simulink model "schemat_8"  (R2020a)
settings: Solver=VariableStepAuto  StartTime=0.0  StopTime=10.0  RelTol=1e-3
values from neighbouring files (symbols this model uses):
  dfwe1 = 0    [gotowe2.m]    (also in lab7.m; lab8.m = 0.5)
  dfwe2 = 0.1*fwemax    (= 0.5)    [gotowe2.m]    (also in lab7.m = 0; lab8.m = 0)
  G11a = A2    (= 10)    [gotowe2.m]    (also in lab8.m)
  G11b = a1+a2    (= 15)    [gotowe2.m]    (also in lab8.m)
  G12 = a1    (= 10)    [gotowe2.m]    (also in lab8.m)
  G21 = a1    (= 10)    [gotowe2.m]    (also in lab8.m)
  G22a = A1    (= 10)    [gotowe2.m]    (also in lab8.m)
  G22b = a1    (= 10)    [gotowe2.m]    (also in lab8.m)
  h10 = (fwe1/a1)+h20    (= 0.8)    [gotowe2.m]    (also in lab7.m = 0.2; lab8.m = (fwe1/a1)+h20)
  h20 = (fwe1+fwe2)/(a2)    (= 0.7)    [gotowe2.m]    (also in lab7.m = 0.2; lab8.m = (fwe1+fwe2)/(a2))
  M1 = A1*A2    (= 100)    [gotowe2.m]    (also in lab8.m)
  M2 = A1*a1+A1*a2+a1*A2    (= 250)    [gotowe2.m]    (also in lab8.m)
  M3 = a1*a2    (= 50)    [gotowe2.m]    (also in lab8.m)
settings Model: Creator=pc  LastModifiedBy=pc

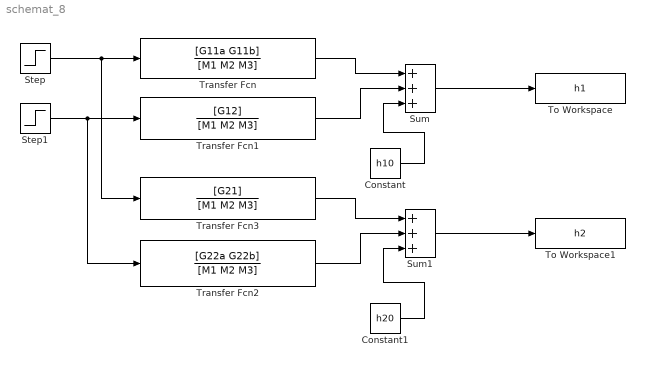
== system schemat_8 ==
  Constant : Constant  Value=h10
  Constant1 : Constant  Value=h20
  Step : Step  Time=5  After=0+dfwe1  SampleTime=0
  Step1 : Step  Time=5  After=0+dfwe2  SampleTime=0
  Sum : Sum  Inputs=+++
  Sum1 : Sum  Inputs=+++
  To Workspace : ToWorkspace  VariableName=h1  SampleTime=-1
  To Workspace1 : ToWorkspace  VariableName=h2  SampleTime=-1
  Transfer Fcn : TransferFcn  Numerator=[G11a G11b]  Denominator=[M1 M2 M3]
  Transfer Fcn1 : TransferFcn  Numerator=[G12]  Denominator=[M1 M2 M3]
  Transfer Fcn2 : TransferFcn  Numerator=[G22a G22b]  Denominator=[M1 M2 M3]
  Transfer Fcn3 : TransferFcn  Numerator=[G21]  Denominator=[M1 M2 M3]
  wires:
  Step/1 -> Transfer Fcn3/1, Transfer Fcn/1
  Step1/1 -> Transfer Fcn2/1, Transfer Fcn1/1
  Transfer Fcn3/1 -> Sum1/1
  Transfer Fcn2/1 -> Sum1/2
  Transfer Fcn/1 -> Sum/1
  Transfer Fcn1/1 -> Sum/2
  Sum/1 -> To Workspace/1
  Sum1/1 -> To Workspace1/1
  Constant/1 -> Sum/3
  Constant1/1 -> Sum1/3
